simulink model "ZeroCross_Detection"  (R2024a)
settings: Solver=FixedStepDiscrete  StartTime=0.0  StopTime=50  FixedStep=1e-6  RelTol=1e-3
libraries: simulink x4
settings Model: Creator=VICTUS  LastModifiedBy=VICTUS

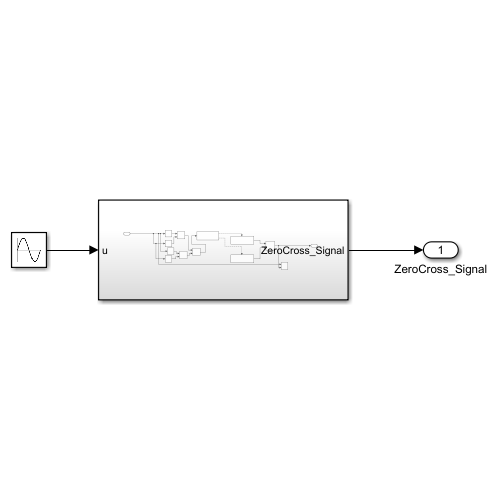
[thumbnail: Simulink's stored preview of the top-level diagram]
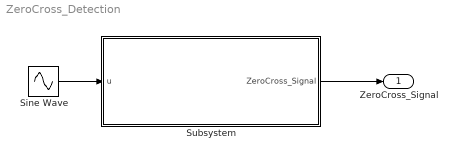
== system ZeroCross_Detection ==
  Sine Wave : Sin  Amplitude=220  SampleTime=0
  Subsystem : Subsystem
  ZeroCross_Signal : Outport
  wires:
  Subsystem/1(ZeroCross_Signal) -> ZeroCross_Signal/1
  Sine Wave/1 -> Subsystem/1(u)

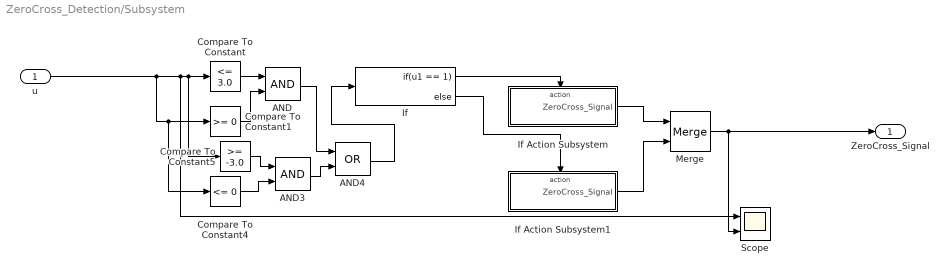
== system ZeroCross_Detection/Subsystem ==
  u : Inport
  AND : Logic  AllPortsSameDT=off  OutDataTypeStr=boolean
  AND3 : Logic  AllPortsSameDT=off  OutDataTypeStr=boolean
  AND4 : Logic  Operator=OR  AllPortsSameDT=off  OutDataTypeStr=boolean
  Compare To Constant : simulink/Logic and Bit Operations/Compare To Constant  relop=<=  const=3.0  OutDataTypeStr=boolean
  Compare To Constant1 : simulink/Logic and Bit Operations/Compare To Constant  relop=>=  const=0  OutDataTypeStr=boolean
  Compare To Constant4 : simulink/Logic and Bit Operations/Compare To Constant  relop=<=  const=0  OutDataTypeStr=boolean
  Compare To Constant5 : simulink/Logic and Bit Operations/Compare To Constant  relop=>=  const=-3.0  OutDataTypeStr=boolean
  If : If  IfExpression=u1 == 1
  If Action Subsystem : Subsystem  TreatAsAtomicUnit=on
  If Action Subsystem1 : Subsystem  TreatAsAtomicUnit=on
  Merge : Merge
  Scope : Scope  NumInputPorts=2
  ZeroCross_Signal : Outport
  wires:
  Compare To Constant1/1 -> AND/2
  u/1 -> Compare To Constant4/1, Compare To Constant1/1, Scope/1, Compare To Constant5/1, Compare To Constant/1
  If Action Subsystem1/1(ZeroCross_Signal) -> Merge/2
  Merge/1 -> ZeroCross_Signal/1, Scope/2
  AND/1 -> AND4/1
  If/2 -> If Action Subsystem1/Action
  Compare To Constant/1 -> AND/1
  If/1 -> If Action Subsystem/Action
  If Action Subsystem/1(ZeroCross_Signal) -> Merge/1
  Compare To Constant4/1 -> AND3/2
  AND3/1 -> AND4/2
  Compare To Constant5/1 -> AND3/1
  AND4/1 -> If/1

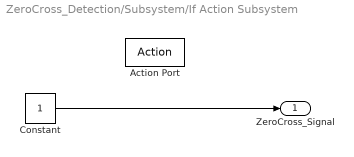
== system ZeroCross_Detection/Subsystem/If Action Subsystem ==
  Action Port : ActionPort  ActionPortLabel=if(u1 == 1)
  Constant : Constant
  ZeroCross_Signal : Outport
  wires:
  Constant/1 -> ZeroCross_Signal/1

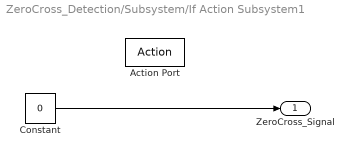
== system ZeroCross_Detection/Subsystem/If Action Subsystem1 ==
  Action Port : ActionPort  ActionPortLabel=else
  Constant : Constant  Value=0
  ZeroCross_Signal : Outport
  wires:
  Constant/1 -> ZeroCross_Signal/1
